simulink model "homework5_2"  (R2021a)
settings: Solver=VariableStepAuto  StartTime=0.0  StopTime=40  RelTol=1e-3
libraries: simulink_extras x4
settings Model: Creator=Godfly  LastModifiedBy=Godfly
settings OptimizationCC: BooleanDataType=off

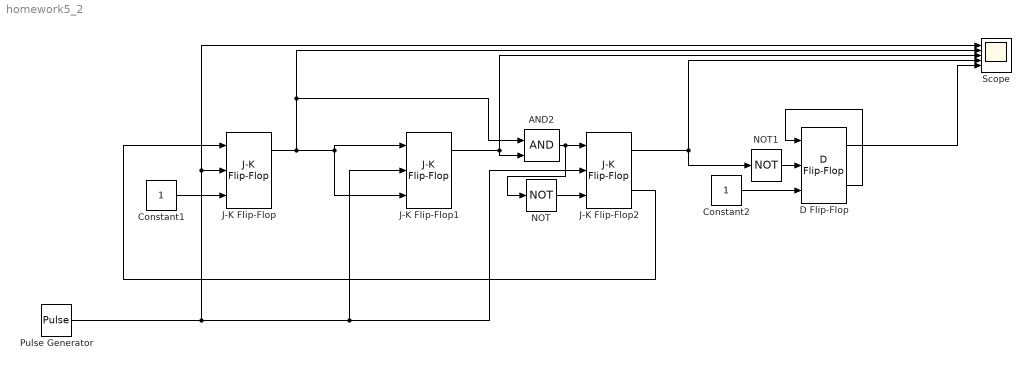
== system homework5_2 ==
  AND2 : Logic  IconShape=distinctive  AllPortsSameDT=off  OutDataTypeStr=boolean
  Constant1 : Constant  OutDataTypeStr=boolean
  Constant2 : Constant  OutDataTypeStr=boolean
  D Flip-Flop : simulink_extras/Flip Flops/D Flip-Flop
  J-K Flip-Flop : simulink_extras/Flip Flops/J-K Flip-Flop  initial_condition=0
  J-K Flip-Flop1 : simulink_extras/Flip Flops/J-K Flip-Flop  initial_condition=0
  J-K Flip-Flop2 : simulink_extras/Flip Flops/J-K Flip-Flop  initial_condition=0
  NOT : Logic  Operator=NOT  IconShape=distinctive  AllPortsSameDT=off  OutDataTypeStr=boolean
  NOT1 : Logic  Operator=NOT  IconShape=distinctive  AllPortsSameDT=off  OutDataTypeStr=boolean
  Pulse Generator : DiscretePulseGenerator  PulseType=Time based  PulseWidth=50  PhaseDelay=1
  Scope : Scope  NumInputPorts=5
  wires:
  J-K Flip-Flop2/2 -> J-K Flip-Flop/1
  J-K Flip-Flop/1 -> J-K Flip-Flop1/3, J-K Flip-Flop1/1, Scope/2, AND2/1
  J-K Flip-Flop1/1 -> Scope/3, AND2/2
  AND2/1 -> NOT/1, J-K Flip-Flop2/1
  Constant1/1 -> J-K Flip-Flop/3
  Pulse Generator/1 -> J-K Flip-Flop2/2, J-K Flip-Flop1/2, Scope/1, J-K Flip-Flop/2
  J-K Flip-Flop2/1 -> NOT1/1, Scope/4
  NOT/1 -> J-K Flip-Flop2/3
  D Flip-Flop/2 -> D Flip-Flop/1
  D Flip-Flop/1 -> Scope/5
  Constant2/1 -> D Flip-Flop/3
  NOT1/1 -> D Flip-Flop/2
